simulink model "PIDmodel2"  (R2013a)
settings: Solver=ode4  StartTime=0.0  StopTime=10.0  FixedStep=0.001  RelTol=1e-3
values from neighbouring files (symbols this model uses):
  ac = 6.250e+00    (= 6.25)    [cdip_para2.m]
  bc = 4.362e+00    (= 4.362)    [cdip_para2.m]
  d = 0    [p1c211_pcont.m]    (also in p1c212_pdcont.m; p1c213_picont.m = -0.1; p1c213_pidcont.m = -0.1; p1c223_pcont.m)
  dtheta_0 = 0    [p1c211_pcont.m]    (also in p1c212_pdcont.m; p1c213_picont.m; p1c213_pidcont.m; p1c221_id_cart.m)
  dz_0 = 0    [p1c211_pcont.m]    (also in p1c212_pdcont.m; p1c213_picont.m; p1c213_pidcont.m; p1c221_id_cart.m)
  kD = 0    [p1c211_pcont.m]    (also in p1c212_pdcont.m = 0.8; p1c213_picont.m; p1c213_pidbode.m = 0.8; p1c213_pidcont.m = 0.8)
  kI = 0    [p1c211_pcont.m]    (also in p1c212_pdcont.m; p1c213_picont.m = 25; p1c213_pidbode.m = 5; p1c213_pidcont.m = 5)
  kP = 20    [p1c211_pcont.m]    (also in p1c212_pdcont.m = 10; p1c213_picont.m = 10; p1c213_pidbode.m = 10; p1c213_pidcont.m = 10)
  omegaM = 10    [p1c223_pcont.m]    (also in p1c224_i_pdcont.m; p1c224_p_dcont.m; p1c23_crane.m)
  ref = 0.1    [p1c211_pcont.m]    (also in p1c212_pdcont.m; p1c213_picont.m; p1c213_pidcont.m; p1c221_id_cart.m = 1.1)
  theta_0 = pi    (= 3.14159265359)    [p1c211_pcont.m]    (also in p1c212_pdcont.m; p1c213_picont.m; p1c213_pidcont.m; p1c221_id_cart.m)
  z_0 = 0    [p1c211_pcont.m]    (also in p1c212_pdcont.m; p1c213_picont.m; p1c213_pidcont.m; p1c221_id_cart.m)
  zetaM = 1/sqrt(2)    [p1c223_pcont.m]    (also in p1c224_p_dcont.m)
undefined symbols (not defined in the file or in its folder): g, Jp, lp, mp, mup
settings Model: Creator=kawata  LastModifiedBy=kawata

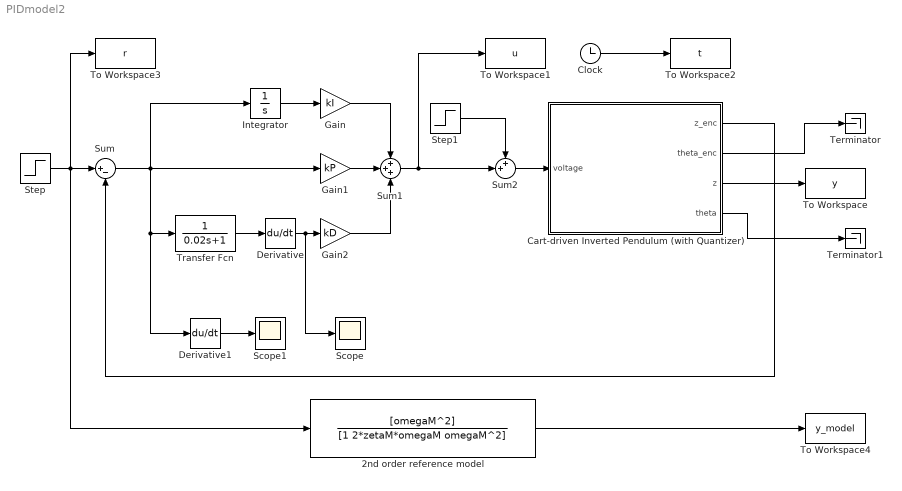
== system PIDmodel2 ==
  2nd order reference model : TransferFcn  Numerator=[omegaM^2]  Denominator=[1 2*zetaM*omegaM omegaM^2]
  Cart-driven Inverted Pendulum (with Quantizer) : Subsystem
      mask Display: image(imread('cdip_photo.jpg'),'center')
  Clock : Clock
  Derivative : Derivative
  Derivative1 : Derivative
  Gain : Gain  Gain=kI
  Gain1 : Gain  Gain=kP
  Gain2 : Gain  Gain=kD
  Integrator : Integrator
  Scope : Scope
  Scope1 : Scope
  Step : Step  Time=0  After=ref  SampleTime=0
  Step1 : Step  Time=0  After=d  SampleTime=0
  Sum : Sum  Inputs=|+-
  Sum1 : Sum  Inputs=+++
  Sum2 : Sum  Inputs=++|
  Terminator : Terminator
  Terminator1 : Terminator
  To Workspace : ToWorkspace  VariableName=y  SampleTime=-1
  To Workspace1 : ToWorkspace  VariableName=u  SampleTime=-1
  To Workspace2 : ToWorkspace  VariableName=t  SampleTime=-1
  To Workspace3 : ToWorkspace  VariableName=r  SampleTime=-1
  To Workspace4 : ToWorkspace  VariableName=y_model  SampleTime=-1
  Transfer Fcn : TransferFcn  Denominator=[0.02 1]
  wires:
  Step/1 -> 2nd order reference model/1, Sum/1, To Workspace3/1
  Gain/1 -> Sum1/1
  Gain1/1 -> Sum1/2
  Gain2/1 -> Sum1/3
  Derivative/1 -> Scope/1, Gain2/1
  Integrator/1 -> Gain/1
  Sum1/1 -> Sum2/2, To Workspace1/1
  Cart-driven Inverted Pendulum (with Quantizer)/1(z_enc) -> Sum/2
  Clock/1 -> To Workspace2/1
  Sum2/1 -> Cart-driven Inverted Pendulum (with Quantizer)/1(voltage)
  Step1/1 -> Sum2/1
  Transfer Fcn/1 -> Derivative/1
  Sum/1 -> Gain1/1, Integrator/1, Transfer Fcn/1, Derivative1/1
  Derivative1/1 -> Scope1/1
  Cart-driven Inverted Pendulum (with Quantizer)/2(theta_enc) -> Terminator/1
  Cart-driven Inverted Pendulum (with Quantizer)/3(z) -> To Workspace/1
  Cart-driven Inverted Pendulum (with Quantizer)/4(theta) -> Terminator1/1
  2nd order reference model/1 -> To Workspace4/1

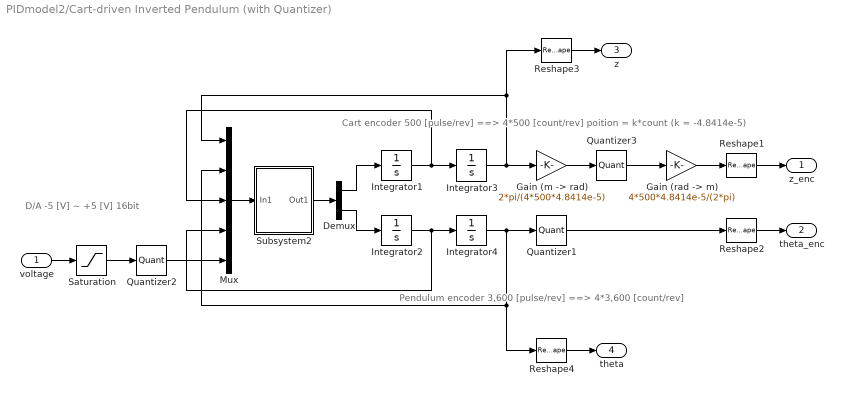
== system PIDmodel2/Cart-driven Inverted Pendulum (with Quantizer) ==
  note: Cart encoder
      |   500 [pulse/rev]  ==> 4*500 [count/rev]
      |   poition = k*count  (k = -4.8414e-5)
  note: D/A
      |   -5 [V] ~ +5 [V]
      |  16bit
  note: Pendulum encoder
      |   3,600 [pulse/rev]  ==> 4*3,600 [count/rev]
  voltage : Inport
  Demux : Demux  Outputs=2
  "Gain (m -> rad)" : Gain  Gain=2*pi/(4*500*4.8414e-5)  SaturateOnIntegerOverflow=on  OutDataTypeStr=Inherit: Same as input  ParamDataTypeStr=Inherit: Same as input
  "Gain (rad -> m)" : Gain  Gain=4*500*4.8414e-5/(2*pi)  SaturateOnIntegerOverflow=on  OutDataTypeStr=Inherit: Same as input  ParamDataTypeStr=Inherit: Same as input
  Integrator1 : Integrator  InitialCondition=dz_0
  Integrator2 : Integrator  InitialCondition=dtheta_0
  Integrator3 : Integrator  InitialCondition=z_0
  Integrator4 : Integrator  InitialCondition=theta_0
  Mux : Mux  Inputs=5
  Quantizer1 : Quantizer  QuantizationInterval=2*pi/(4*3600)
  Quantizer2 : Quantizer  QuantizationInterval=10/2^(16)
  Quantizer3 : Quantizer  QuantizationInterval=2*pi/(4*500)
  Reshape{1..4} (4 alike) : Reshape
  Saturation : Saturate  UpperLimit=5  LowerLimit=-5
  Subsystem2 : Subsystem
  z_enc : Outport
  theta_enc : Outport  Port=2
  z : Outport  Port=3
  theta : Outport  Port=4
  wires:
  Reshape4/1 -> theta/1
  Reshape3/1 -> z/1
  Saturation/1 -> Quantizer2/1
  Quantizer2/1 -> Mux/5
  Quantizer1/1 -> Reshape2/1
  Subsystem2/1(Out1) -> Demux/1
  Mux/1 -> Subsystem2/1(In1)
  Demux/1 -> Integrator1/1
  Demux/2 -> Integrator2/1
  Integrator1/1 -> Mux/3, Integrator3/1
  Integrator2/1 -> Mux/4, Integrator4/1
  Integrator3/1 -> Reshape3/1, Mux/1, "Gain (m -> rad)"/1
  Integrator4/1 -> Reshape4/1, Mux/2, Quantizer1/1
  voltage/1 -> Saturation/1
  "Gain (m -> rad)"/1 -> Quantizer3/1
  Quantizer3/1 -> "Gain (rad -> m)"/1
  "Gain (rad -> m)"/1 -> Reshape1/1
  Reshape1/1 -> z_enc/1
  Reshape2/1 -> theta_enc/1

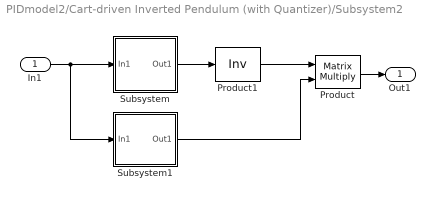
== system PIDmodel2/Cart-driven Inverted Pendulum (with Quantizer)/Subsystem2 ==
  In1 : Inport
  Product : Product  Multiplication=Matrix(*)  SaturateOnIntegerOverflow=on  InputSameDT=on  OutDataTypeStr=Inherit: Same as first input
  Product1 : Product  Inputs=/  Multiplication=Matrix(*)  SaturateOnIntegerOverflow=on  InputSameDT=on  OutDataTypeStr=Inherit: Same as first input
  Subsystem : Subsystem
  Subsystem1 : Subsystem
  Out1 : Outport
  wires:
  Subsystem/1(Out1) -> Product1/1
  Product1/1 -> Product/1
  Subsystem1/1(Out1) -> Product/2
  In1/1 -> Subsystem/1(In1), Subsystem1/1(In1)
  Product/1 -> Out1/1

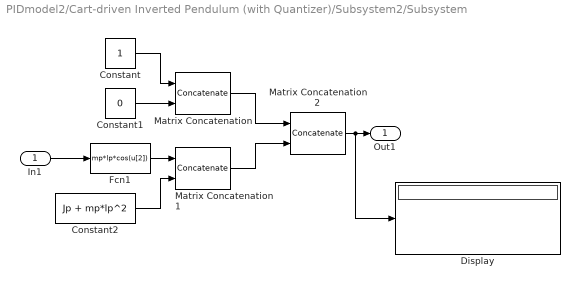
== system PIDmodel2/Cart-driven Inverted Pendulum (with Quantizer)/Subsystem2/Subsystem ==
  In1 : Inport
  Constant : Constant
  Constant1 : Constant  Value=0
  Constant2 : Constant  Value=Jp + mp*lp^2
  Display : Display
  Fcn1 : Fcn  Expr=mp*lp*cos(u[2])
  Matrix Concatenation : Concatenate  Mode=Multidimensional array  ConcatenateDimension=2
  Matrix Concatenation1 : Concatenate  Mode=Multidimensional array  ConcatenateDimension=2
  Matrix Concatenation2 : Concatenate  Mode=Multidimensional array
  Out1 : Outport
  wires:
  Constant2/1 -> Matrix Concatenation1/2
  Fcn1/1 -> Matrix Concatenation1/1
  In1/1 -> Fcn1/1
  Matrix Concatenation/1 -> Matrix Concatenation2/1
  Matrix Concatenation1/1 -> Matrix Concatenation2/2
  Matrix Concatenation2/1 -> Display/1, Out1/1
  Constant/1 -> Matrix Concatenation/1
  Constant1/1 -> Matrix Concatenation/2

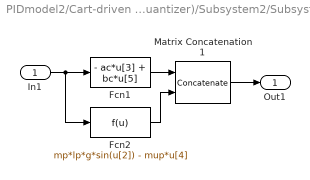
== system PIDmodel2/Cart-driven Inverted Pendulum (with Quantizer)/Subsystem2/Subsystem1 ==
  In1 : Inport
  Fcn1 : Fcn  Expr=- ac*u[3] + bc*u[5]
  Fcn2 : Fcn  Expr=mp*lp*g*sin(u[2]) - mup*u[4]
  Matrix Concatenation1 : Concatenate  Mode=Multidimensional array
  Out1 : Outport
  wires:
  Fcn2/1 -> Matrix Concatenation1/2
  Fcn1/1 -> Matrix Concatenation1/1
  In1/1 -> Fcn2/1, Fcn1/1
  Matrix Concatenation1/1 -> Out1/1
